simulink model "ASM"  (R2014a)
settings: Solver=ode45  StartTime=0.0  StopTime=30  FixedStep=0.002  MaxStep=0.2e-3  RelTol=1e-3
PreLoadFcn:
  | ASM_init
model workspace: external: MATLAB File /Users/Pascal/Documents/Beuth Hochschule/EPE-MES/04_Simulation/ASM/ASM_init.m (data not in the file)
values from neighbouring files (symbols this model uses):
  J = 0.0006    [ASM_init.m]    (also in parameter.mat)
  LR_plus = 0.89737    [ASM_init.m]    (also in parameter.mat)
  Lsigma_plus = 0.12968    [ASM_init.m]    (also in parameter.mat)
  MLast = 2    [ASM_init.m]    (also in parameter.mat = 20)
  MLast1 = 3.8    [ASM_init.m]
  PsiR_plus = 0.64521    [ASM_init.m]    (also in parameter.mat)
  RR_plus = 26.3    [ASM_init.m]    (also in parameter.mat)
  Rreib = 0.00138    [ASM_init.m]    (also in parameter.mat = 0.16)
  Rs = 32.65    [ASM_init.m]    (also in parameter.mat)
  wSoll = 500    [ASM_init.m]
  wSoll2 = 200    [ASM_init.m]
libraries: powerlib x25, simulink x3
settings Model: SimulationMode=accelerator  Creator=Pascal  LastModifiedBy=Pascal
settings DataIOCC: ExternalInput=parameter.mat  FinalStateName=ASM_state  InitialState=ASM_state  LimitDataPoints=off  SaveCompleteFinalSimState=on  SaveOutput=off
settings HardwareCC: ProdBitPerChar=16  ProdBitPerInt=16  ProdBitPerPointer=16  ProdLargestAtomicInteger=Integer  ProdIntDivRoundTo=Zero  ProdEndianess=LittleEndian  ProdWordSize=16  ProdHWDeviceType=Texas Instruments->C2000

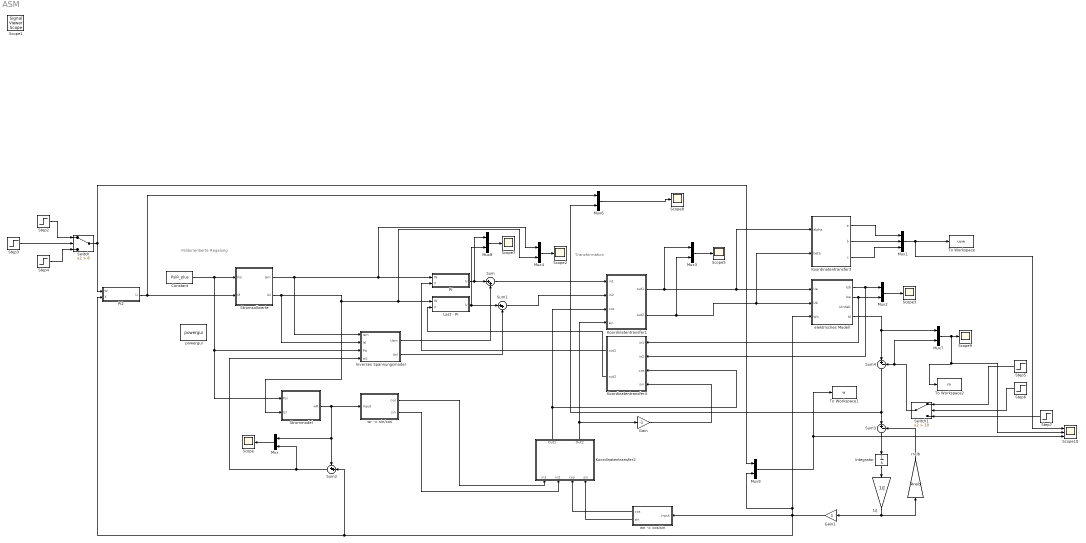
== system ASM ==
  note: Transformation
  note: Feldorientierte Regelung
  1/J : Gain  Gain=1/J
  Constant : Constant  Value=PsiR_plus
  Gain : Gain  Gain=-1
  Gain1 : Gain
  Integrator : Integrator
  "Inverses Spannungsmodel " : Subsystem
  Koordinatentransfer1 : Subsystem
  Koordinatentransfer2 : Subsystem
  Koordinatentransfer3 : Subsystem
  Koordinatentransfer4 : Subsystem
  Last - PI : Subsystem
  Mux{,2..4,6..9} (8 alike) : Mux  Inputs=2
  Mux1 : Mux  Inputs=3
  PI : Subsystem
  PI2 : Subsystem
  Scope{,2..3,5,7..9} (7 alike) : Scope
      Scope settings: ShowLegends=on  TimeRange=1  YMin=200  YMax=1500  SaveName=ScopeData6
      Scope2 settings: ShowLegends=on  TimeRange=4  YMin=-0.325  YMax=0.15
      Scope3 settings: ShowLegends=on  YMin=5000  YMax=70000  SaveName=ScopeData9
      Scope5 settings: YMin=-900  YMax=900
      Scope7 settings: ShowLegends=on  TimeRange=4  YMin=120  YMax=330  SaveName=ScopeData3
      Scope8 settings: ShowLegends=on  YMin=1  YMax=1.8  SaveName=ScopeData4
      Scope9 settings: ShowLegends=on  YMin=1.38778e-17  YMax=0.3  SaveName=ScopeData7
  Scope10 : Scope  NumInputPorts=3
      settings: ShowLegends=on  TimeRange=4  YMin=-1500~0~1350  YMax=1500~2~1420  SaveName=ScopeData10
  Step2 : Step  Before=1350  After=wSoll  SampleTime=0
  Step3 : Step  Time=8  After=200  SampleTime=0
  Step4 : Step  Time=3  Before=1350  After=wSoll2  SampleTime=0
  Step5 : Step  Time=4  After=MLast  SampleTime=0
  Step6 : Step  Time=10  After=200  SampleTime=0
  Step7 : Step  Time=3  After=MLast1  SampleTime=0
  "Strommodel " : Subsystem
  Stromsollwerte : Subsystem
  Sum : Sum  Inputs=|++
  Sum1 : Sum  Inputs=|++
  Sum2 : Sum  Inputs=++|
  Sum3 : Sum  Inputs=|+-
  Sum4 : Sum  Inputs=|+-
  Switch : Switch  Criteria=u2 > Threshold  Threshold=8
  Switch1 : Switch  Criteria=u2 > Threshold  Threshold=10
  To Workspace : ToWorkspace  VariableName=uvw  SampleTime=-1
  To Workspace1 : ToWorkspace  VariableName=w  SampleTime=-1
  To Workspace2 : ToWorkspace  VariableName=m  SampleTime=-1
  elektrisches Modell : Subsystem
  powergui : powerlib/powergui  Priority=1  SimulationMode=Continuous  SolverType=Tustin  SampleTime=50e-6  frequency=60  SPID=off  DisableSnubberDevices=off  DisableRonSwitches=off  DisableVfSwitches=off  SwTol=0  Interpol=off  DisplayEquations=off  Ts=0  methode=off  frequencyindice=0  Pbase=100e6  ErrMax=1e-4  Iterations=50  UnitsV=kV  UnitsW=MW  FunctionMessages=off  echomessages=off  HookPort=off  EnableUseOfTLC=off  x0status=blocks  RestoreLinks=warning  ResistiveCurrentMeasurement=off  Frange=[0:2:500]  Ylog=off  Xlog=on  ShowGrid=off  save=off  variable=ZData  structure=0  ZoomFFT=off  StartTime=0.0  cycles=1  DisplayStyle=1  fundamental=60  FreqAxis=off  MaxFrequency=1000  frequencyindicesteady=1  RmsSteady=1  display=off
  rreib : Gain  Gain=Rreib
  "wn -> cos/sin" : Subsystem
  "wr -> sin/cos" : Subsystem
  Scope1 : SignalViewerScope  IOType=viewer  ZoomMode=xonly  RefreshTime=0.035000
  wires:
  Mux2/1 -> Scope3/1
  Koordinatentransfer2/2(Out2) -> Gain/1, Koordinatentransfer1/4(sin)
  "wn -> cos/sin"/1(cos) -> Koordinatentransfer2/3(cos)
  "Strommodel "/1(wR) -> Sum2/1, Mux/1, "wr -> sin/cos"/1(Input)
  "wn -> cos/sin"/2(sin) -> Koordinatentransfer2/4("sin ")
  "wr -> sin/cos"/1(cos) -> Koordinatentransfer2/1(in1)
  Sum2/1 -> Mux/2, "Inverses Spannungsmodel "/4(wS)
  PI/1(U) -> Mux8/1, Sum/1
  Koordinatentransfer2/1(Out1) -> Koordinatentransfer1/3(cos), Koordinatentransfer4/3(cos)
  "wr -> sin/cos"/2(sin) -> Koordinatentransfer2/2(in2)
  Last - PI/1(U) -> Mux8/2, Sum1/1
  elektrisches Modell/1(Isb) -> Koordinatentransfer4/2(in2), Mux2/1
  elektrisches Modell/2(Isa) -> Koordinatentransfer4/1(in1), Mux2/2
  Koordinatentransfer3/2(b) -> Mux1/2
  Koordinatentransfer3/1(a) -> Mux1/1
  Koordinatentransfer3/3(c) -> Mux1/3
  1/J/1 -> rreib/1, Gain1/1
  Mux3/1 -> Scope5/1
  Constant/1 -> "Strommodel "/1(Psi), "Inverses Spannungsmodel "/3(Psi), Stromsollwerte/1(Psi)
  Gain/1 -> Koordinatentransfer4/4(sin)
  Sum3/1 -> Integrator/1
  rreib/1 -> Sum3/2
  Integrator/1 -> 1/J/1
  Sum4/1 -> Mux6/2, Sum3/1
  Mux6/1 -> Scope8/1
  Mux/1 -> Scope/1
  Mux7/1 -> To Workspace2/1, Scope10/2, Scope9/1
  elektrisches Modell/4(M) -> Mux7/1, Sum4/1
  Switch1/1 -> Mux7/2, Sum4/2
  Stromsollwerte/1(Ism) -> Mux4/1, PI/1(W), "Inverses Spannungsmodel "/1(Ism)
  Stromsollwerte/2(Isl) -> "Inverses Spannungsmodel "/2(Isl), "Strommodel "/2(Isl), Mux4/2, Last - PI/1(W)
  Koordinatentransfer4/2(out2) -> Last - PI/2(X)
  Koordinatentransfer4/1(out1) -> PI/2(X)
  Step2/1 -> Switch/1
  Mux1/1 -> Scope10/1, To Workspace/1
  Mux9/1 -> Scope10/3, To Workspace1/1
  Switch/1 -> PI2/1(W), Mux9/1
  Step4/1 -> Switch/3
  Step3/1 -> Switch/2
  Koordinatentransfer1/2(out2) -> Mux3/2, elektrisches Modell/2(Ub), Koordinatentransfer3/2(beta)
  Koordinatentransfer1/1(out1) -> elektrisches Modell/1(Ua), Koordinatentransfer3/1(alpha), Mux3/1
  Mux8/1 -> Scope7/1
  Mux4/1 -> Scope2/1
  "Inverses Spannungsmodel "/1(Usm) -> Sum/2
  "Inverses Spannungsmodel "/2(Usl) -> Sum1/2
  Sum/1 -> Koordinatentransfer1/1(in1)
  Sum1/1 -> Koordinatentransfer1/2(in2)
  Gain1/1 -> Mux9/2, elektrisches Modell/3(Wn), "wn -> cos/sin"/1(Input), PI2/2(X), Sum2/2
  PI2/1(U) -> Stromsollwerte/2(M), Mux6/1
  Step5/1 -> Switch1/1
  Step7/1 -> Switch1/3
  Step6/1 -> Switch1/2

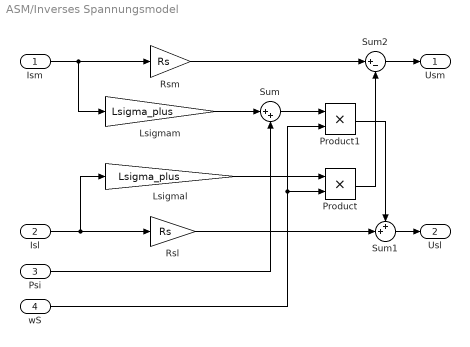
== system ASM/Inverses Spannungsmodel  ==
  Ism : Inport
  Isl : Inport  Port=2
  Psi : Inport  Port=3
  wS : Inport  Port=4
  Lsigmal : Gain  Gain=Lsigma_plus
  Lsigmam : Gain  Gain=Lsigma_plus
  Product : Product
  Product1 : Product
  Rsl : Gain  Gain=Rs
  Rsm : Gain  Gain=Rs
  Sum : Sum  Inputs=|++
  Sum1 : Sum  Inputs=++|
  Sum2 : Sum  Inputs=|+-
  Usm : Outport
  Usl : Outport  Port=2
  wires:
  Lsigmam/1 -> Sum/1
  Ism/1 -> Rsm/1, Lsigmam/1
  Isl/1 -> Rsl/1, Lsigmal/1
  Sum2/1 -> Usm/1
  Sum1/1 -> Usl/1
  Sum/1 -> Product1/1
  wS/1 -> Product1/2, Product/2
  Lsigmal/1 -> Product/1
  Psi/1 -> Sum/2
  Product1/1 -> Sum1/1
  Product/1 -> Sum2/2
  Rsm/1 -> Sum2/1
  Rsl/1 -> Sum1/2

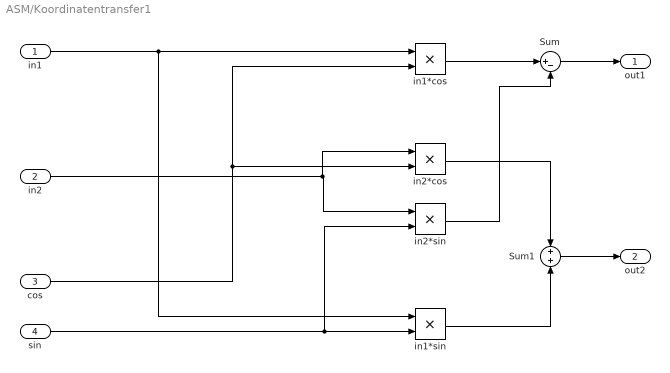
== system ASM/Koordinatentransfer1 ==
  in1 : Inport
  in2 : Inport  Port=2
  cos : Inport  Port=3
  sin : Inport  Port=4
  Sum : Sum  Inputs=|+-
  Sum1 : Sum
  in1*cos : Product
  in1*sin : Product
  in2*cos : Product
  in2*sin : Product
  out1 : Outport
  out2 : Outport  Port=2
  wires:
  in1/1 -> in1*sin/1, in1*cos/1
  cos/1 -> in2*cos/2, in1*cos/2
  sin/1 -> in2*sin/2, in1*sin/2
  in2/1 -> in2*cos/1, in2*sin/1
  in1*sin/1 -> Sum1/2
  in2*cos/1 -> Sum1/1
  in2*sin/1 -> Sum/2
  in1*cos/1 -> Sum/1
  Sum/1 -> out1/1
  Sum1/1 -> out2/1

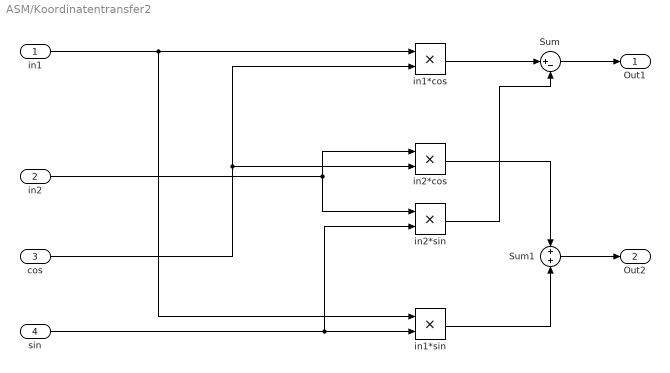
== system ASM/Koordinatentransfer2 ==
  in1 : Inport
  in2 : Inport  Port=2
  cos : Inport  Port=3
  "sin " : Inport  Port=4
  Sum : Sum  Inputs=|+-
  Sum1 : Sum
  in1*cos : Product
  in1*sin : Product
  in2*cos : Product
  in2*sin : Product
  Out1 : Outport
  Out2 : Outport  Port=2
  wires:
  in1/1 -> in1*sin/1, in1*cos/1
  cos/1 -> in2*cos/2, in1*cos/2
  "sin "/1 -> in2*sin/2, in1*sin/2
  in2/1 -> in2*cos/1, in2*sin/1
  in1*sin/1 -> Sum1/2
  in2*cos/1 -> Sum1/1
  in2*sin/1 -> Sum/2
  in1*cos/1 -> Sum/1
  Sum/1 -> Out1/1
  Sum1/1 -> Out2/1

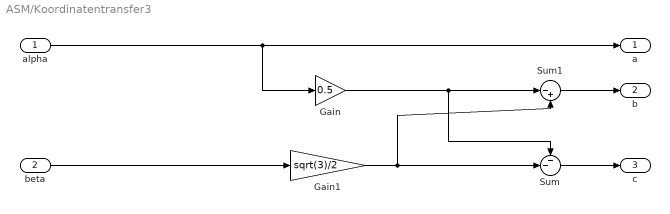
== system ASM/Koordinatentransfer3 ==
  alpha : Inport
  beta : Inport  Port=2
  Gain : Gain  Gain=0.5
  Gain1 : Gain  Gain=sqrt(3)/2
  Sum : Sum  Inputs=--|
  Sum1 : Sum  Inputs=|-+
  a : Outport
  b : Outport  Port=2
  c : Outport  Port=3
  wires:
  alpha/1 -> Gain/1, a/1
  Sum1/1 -> b/1
  Gain/1 -> Sum/1, Sum1/1
  Gain1/1 -> Sum/2, Sum1/2
  beta/1 -> Gain1/1
  Sum/1 -> c/1

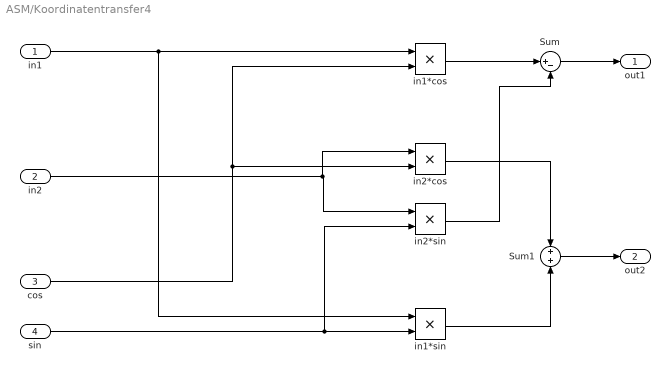
== system ASM/Koordinatentransfer4 ==
  in1 : Inport
  in2 : Inport  Port=2
  cos : Inport  Port=3
  sin : Inport  Port=4
  Sum : Sum  Inputs=|+-
  Sum1 : Sum
  in1*cos : Product
  in1*sin : Product
  in2*cos : Product
  in2*sin : Product
  out1 : Outport
  out2 : Outport  Port=2
  wires:
  in1/1 -> in1*sin/1, in1*cos/1
  cos/1 -> in2*cos/2, in1*cos/2
  sin/1 -> in2*sin/2, in1*sin/2
  in2/1 -> in2*cos/1, in2*sin/1
  in1*sin/1 -> Sum1/2
  in2*cos/1 -> Sum1/1
  in2*sin/1 -> Sum/2
  in1*cos/1 -> Sum/1
  Sum/1 -> out1/1
  Sum1/1 -> out2/1

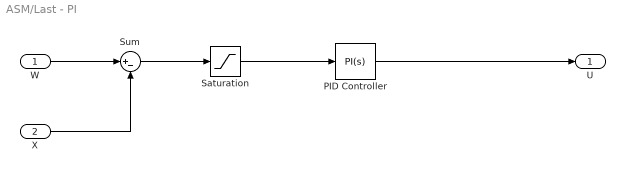
== system ASM/Last - PI ==
  W : Inport
  X : Inport  Port=2
  PID Controller : simulink/Continuous/PID Controller  Controller=PI  TimeDomain=Continuous-time  SampleTime=1  IntegratorMethod=Forward Euler  FilterMethod=Forward Euler  Form=Parallel  P=3.02729379594108  I=59.0597737641669  D=0.0225096512911581  N=2097943.11620465  InitialConditionSource=internal  InitialConditionForIntegrator=0  InitialConditionForFilter=0  ExternalReset=none  LimitOutput=on  UpperSaturationLimit=325  LowerSaturationLimit=-325  LinearizeAsGain=off  AntiWindupMode=none  Kb=1  TrackingMode=off  Kt=1  PParamMin=[]  PParamMax=[]  IParamMin=[]  IParamMax=[]  DParamMin=[]  DParamMax=[]  NParamMin=[]  NParamMax=[]  KbParamMin=[]  KbParamMax=[]  KtParamMin=[]  KtParamMax=[]  POutMin=[]  POutMax=[]  IOutMin=[]  IOutMax=[]  DOutMin=[]  DOutMax=[]  NOutMin=[]  NOutMax=[]  KbOutMin=[]  KbOutMax=[]  KtOutMin=[]  KtOutMax=[]  IntegratorOutMin=[]  IntegratorOutMax=[]  FilterOutMin=[]  FilterOutMax=[]  SumOutMin=[]  SumOutMax=[]  SumI1OutMin=[]  SumI1OutMax=[]  SumI2OutMin=[]  SumI2OutMax=[]  SumI3OutMin=[]  SumI3OutMax=[]  SumDOutMin=[]  SumDOutMax=[]  SaturationOutMin=[]  SaturationOutMax=[]  IntegratorContinuousStateAttributes=''  IntegratorStateMustResolveToSignalObject=off  IntegratorRTWStateStorageClass=Auto  FilterContinuousStateAttributes=''  FilterStateMustResolveToSignalObject=off  FilterRTWStateStorageClass=Auto
  Saturation : Saturate  UpperLimit=3.8  LowerLimit=-3.8  LinearizeAsGain=off
  Sum : Sum  Inputs=|+-
  U : Outport
  wires:
  W/1 -> Sum/1
  X/1 -> Sum/2
  Sum/1 -> Saturation/1
  PID Controller/1 -> U/1
  Saturation/1 -> PID Controller/1

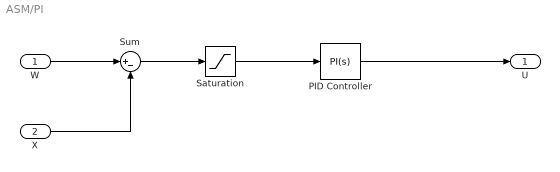
== system ASM/PI ==
  W : Inport
  X : Inport  Port=2
  PID Controller : simulink/Continuous/PID Controller  Controller=PI  TimeDomain=Continuous-time  SampleTime=1  IntegratorMethod=Forward Euler  FilterMethod=Forward Euler  Form=Parallel  P=3.02729379594108  I=59.0597737641669  D=0.0225096512911581  N=2097943.11620465  InitialConditionSource=internal  InitialConditionForIntegrator=0  InitialConditionForFilter=0  ExternalReset=none  LimitOutput=on  UpperSaturationLimit=325  LowerSaturationLimit=-325  LinearizeAsGain=off  AntiWindupMode=none  Kb=1  TrackingMode=off  Kt=1  PParamMin=[]  PParamMax=[]  IParamMin=[]  IParamMax=[]  DParamMin=[]  DParamMax=[]  NParamMin=[]  NParamMax=[]  KbParamMin=[]  KbParamMax=[]  KtParamMin=[]  KtParamMax=[]  POutMin=[]  POutMax=[]  IOutMin=[]  IOutMax=[]  DOutMin=[]  DOutMax=[]  NOutMin=[]  NOutMax=[]  KbOutMin=[]  KbOutMax=[]  KtOutMin=[]  KtOutMax=[]  IntegratorOutMin=[]  IntegratorOutMax=[]  FilterOutMin=[]  FilterOutMax=[]  SumOutMin=[]  SumOutMax=[]  SumI1OutMin=[]  SumI1OutMax=[]  SumI2OutMin=[]  SumI2OutMax=[]  SumI3OutMin=[]  SumI3OutMax=[]  SumDOutMin=[]  SumDOutMax=[]  SaturationOutMin=[]  SaturationOutMax=[]  IntegratorContinuousStateAttributes=''  IntegratorStateMustResolveToSignalObject=off  IntegratorRTWStateStorageClass=Auto  FilterContinuousStateAttributes=''  FilterStateMustResolveToSignalObject=off  FilterRTWStateStorageClass=Auto
  Saturation : Saturate  UpperLimit=3.8  LowerLimit=-3.8  LinearizeAsGain=off
  Sum : Sum  Inputs=|+-
  U : Outport
  wires:
  W/1 -> Sum/1
  X/1 -> Sum/2
  Sum/1 -> Saturation/1
  PID Controller/1 -> U/1
  Saturation/1 -> PID Controller/1

== system ASM/PI2 ==
  W : Inport
  X : Inport  Port=2
  PID Controller : simulink/Continuous/PID Controller  Controller=PI  TimeDomain=Continuous-time  SampleTime=1  IntegratorMethod=Forward Euler  FilterMethod=Forward Euler  Form=Parallel  P=0.0785257439463388  I=0.0278541269001317  D=0  N=1000  InitialConditionSource=internal  InitialConditionForIntegrator=0  InitialConditionForFilter=0  ExternalReset=none  LimitOutput=on  UpperSaturationLimit=3.4  LowerSaturationLimit=-3.4  LinearizeAsGain=off  AntiWindupMode=none  Kb=1  TrackingMode=off  Kt=1  PParamMin=[]  PParamMax=[]  IParamMin=[]  IParamMax=[]  DParamMin=[]  DParamMax=[]  NParamMin=[]  NParamMax=[]  KbParamMin=[]  KbParamMax=[]  KtParamMin=[]  KtParamMax=[]  POutMin=[]  POutMax=[]  IOutMin=[]  IOutMax=[]  DOutMin=[]  DOutMax=[]  NOutMin=[]  NOutMax=[]  KbOutMin=[]  KbOutMax=[]  KtOutMin=[]  KtOutMax=[]  IntegratorOutMin=[]  IntegratorOutMax=[]  FilterOutMin=[]  FilterOutMax=[]  SumOutMin=[]  SumOutMax=[]  SumI1OutMin=[]  SumI1OutMax=[]  SumI2OutMin=[]  SumI2OutMax=[]  SumI3OutMin=[]  SumI3OutMax=[]  SumDOutMin=[]  SumDOutMax=[]  SaturationOutMin=[]  SaturationOutMax=[]  IntegratorContinuousStateAttributes=''  IntegratorStateMustResolveToSignalObject=off  IntegratorRTWStateStorageClass=Auto  FilterContinuousStateAttributes=''  FilterStateMustResolveToSignalObject=off  FilterRTWStateStorageClass=Auto
  Sum : Sum  Inputs=|+-
  U : Outport
  wires:
  W/1 -> Sum/1
  X/1 -> Sum/2
  PID Controller/1 -> U/1
  Sum/1 -> PID Controller/1

== system ASM/Strommodel  ==
  Psi : Inport
  Isl : Inport  Port=2
  Divide : Product  Inputs=*/
  Rr : Gain  Gain=RR_plus
  wR : Outport
  wires:
  Rr/1 -> wR/1
  Divide/1 -> Rr/1
  Psi/1 -> Divide/2
  Isl/1 -> Divide/1

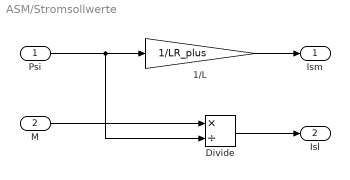
== system ASM/Stromsollwerte ==
  Psi : Inport
  M : Inport  Port=2
  1/L : Gain  Gain=1/LR_plus
  Divide : Product  Inputs=*/
  Ism : Outport  OutMax=1.8
  Isl : Outport  Port=2  OutMax=[1.8]
  wires:
  1/L/1 -> Ism/1
  Psi/1 -> Divide/2, 1/L/1
  Divide/1 -> Isl/1
  M/1 -> Divide/1

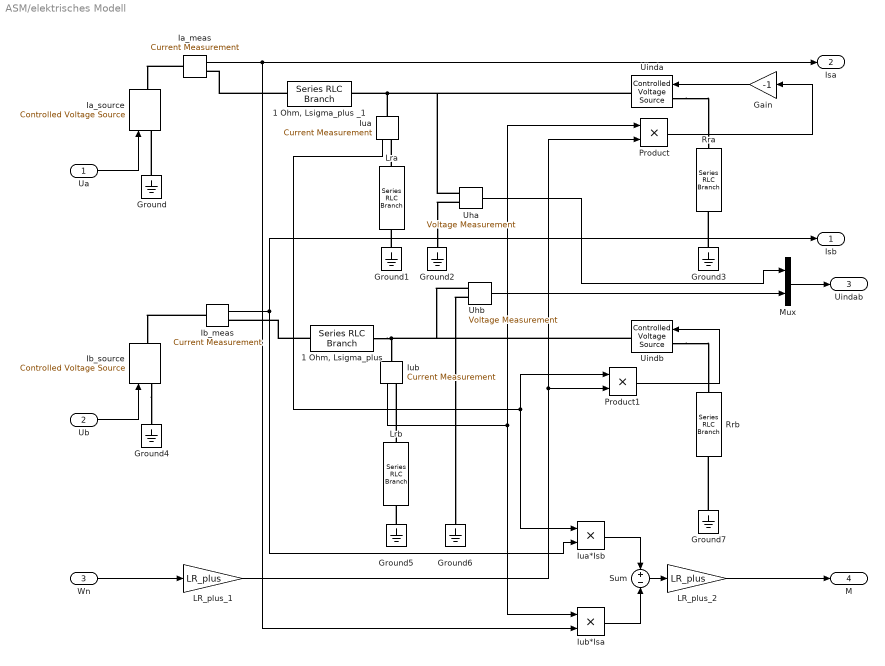
== system ASM/elektrisches Modell ==
  Ua : Inport
  Ub : Inport  Port=2
  Wn : Inport  Port=3
  "1 Ohm, Lsigma_plus" : powerlib/Elements/Series RLC Branch  LConnTagsString=__new0  RConnTagsString=__new0  BranchType=RL  Resistance=RR_plus  Inductance=Lsigma_plus  SetiL0=on  InitialCurrent=10  Capacitance=1e-6  Setx0=off  InitialVoltage=0  Measurements=None
  "1 Ohm, Lsigma_plus _1 " : powerlib/Elements/Series RLC Branch  LConnTagsString=__new0  RConnTagsString=__new0  BranchType=RL  Resistance=RR_plus  Inductance=Lsigma_plus  SetiL0=on  InitialCurrent=10  Capacitance=1e-6  Setx0=off  InitialVoltage=0  Measurements=None
  Gain : Gain  Gain=-1
  Ground{,1..7} (8 alike) : powerlib/Elements/Ground  LConnTagsString=a
  Ia_meas : powerlib/Measurements/Current Measurement  PhasorSimulation=off  OutputType=Complex  PSBequivalent=0
  Ia_source : powerlib/Electrical Sources/Controlled Voltage Source  Initialize=on  Source_Type=AC  Amplitude=0  Phase=0  Frequency=0  Measurements=None
  Ib_meas : powerlib/Measurements/Current Measurement  PhasorSimulation=off  OutputType=Complex  PSBequivalent=0
  Ib_source : powerlib/Electrical Sources/Controlled Voltage Source  Initialize=on  Source_Type=AC  Amplitude=0  Phase=0  Frequency=0  Measurements=None
  Iua : powerlib/Measurements/Current Measurement  PhasorSimulation=off  OutputType=Complex  PSBequivalent=0
  Iua*Isb : Product
  Iub : powerlib/Measurements/Current Measurement  PhasorSimulation=off  OutputType=Complex  PSBequivalent=0
  Iub*Isa : Product
  LR_plus_1 : Gain  Gain=LR_plus
  LR_plus_2 : Gain  Gain=LR_plus
  Lra : powerlib/Elements/Series RLC Branch  LConnTagsString=__new0  RConnTagsString=__new0  BranchType=L  Resistance=1  Inductance=LR_plus  SetiL0=on  InitialCurrent=10  Capacitance=1e-6  Setx0=off  InitialVoltage=0  Measurements=None
  Lrb : powerlib/Elements/Series RLC Branch  LConnTagsString=__new0  RConnTagsString=__new0  BranchType=L  Resistance=1  Inductance=LR_plus  SetiL0=on  InitialCurrent=10  Capacitance=1e-6  Setx0=off  InitialVoltage=0  Measurements=None
  Mux : Mux  Inputs=2
  Product : Product
  Product1 : Product
  Rra : powerlib/Elements/Series RLC Branch  LConnTagsString=__new0  RConnTagsString=__new0  BranchType=R  Resistance=RR_plus  Inductance=100e-3  SetiL0=off  InitialCurrent=0  Capacitance=1e-6  Setx0=off  InitialVoltage=0  Measurements=None
  Rrb : powerlib/Elements/Series RLC Branch  LConnTagsString=__new0  RConnTagsString=__new0  BranchType=R  Resistance=RR_plus  Inductance=100e-3  SetiL0=off  InitialCurrent=0  Capacitance=1e-6  Setx0=off  InitialVoltage=0  Measurements=None
  Sum : Sum  Inputs=+|-
  Uha : powerlib/Measurements/Voltage Measurement  PhasorSimulation=off  OutputType=Complex  PSBequivalent=0
  Uhb : powerlib/Measurements/Voltage Measurement  PhasorSimulation=off  OutputType=Complex  PSBequivalent=0
  Uinda : powerlib/Electrical Sources/Controlled Voltage Source  Initialize=on  Source_Type=AC  Amplitude=0  Phase=0  Frequency=0  Measurements=None
  Uindb : powerlib/Electrical Sources/Controlled Voltage Source  Initialize=on  Source_Type=AC  Amplitude=0  Phase=0  Frequency=0  Measurements=None
  Isb : Outport
  Isa : Outport  Port=2
  Uindab : Outport  Port=3
  M : Outport  Port=4
  wires:
  Ua/1 -> Ia_source/1
  Ia_meas/1 -> Iub*Isa/2, Isa/1
  Gain/1 -> Uinda/1
  Product/1 -> Gain/1
  Ub/1 -> Ib_source/1
  Ib_meas/1 -> Iua*Isb/2, Isb/1
  Uhb/1 -> Mux/2
  Uha/1 -> Mux/1
  Iub/1 -> Iub*Isa/1, Product/1
  Product1/1 -> Uindb/1
  Iua/1 -> Product1/1, Iua*Isb/1
  Wn/1 -> LR_plus_1/1
  LR_plus_1/1 -> Product/2, Product1/2
  Mux/1 -> Uindab/1
  Sum/1 -> LR_plus_2/1
  Iub*Isa/1 -> Sum/2
  Iua*Isb/1 -> Sum/1
  LR_plus_2/1 -> M/1
  connections:
  Ground/LConn1 -- Ia_source/LConn1
  Ia_meas/LConn1 -- Ia_source/RConn1
  "1 Ohm, Lsigma_plus _1 "/LConn1 -- Ia_meas/RConn1
  Iua/LConn1 -- Uha/LConn1 -- Uinda/RConn1 -- "1 Ohm, Lsigma_plus _1 "/RConn1
  Lra/LConn1 -- Iua/RConn1
  Ground1/LConn1 -- Lra/RConn1
  Uha/LConn2 -- Ground2/LConn1
  Uinda/LConn1 -- Rra/LConn1
  Ground3/LConn1 -- Rra/RConn1
  Ib_source/LConn1 -- Ground4/LConn1
  Ib_meas/LConn1 -- Ib_source/RConn1
  "1 Ohm, Lsigma_plus"/LConn1 -- Ib_meas/RConn1
  Lrb/LConn1 -- Iub/RConn1
  Ground5/LConn1 -- Lrb/RConn1
  Uhb/LConn2 -- Ground6/LConn1
  "1 Ohm, Lsigma_plus"/RConn1 -- Uindb/RConn1 -- Uhb/LConn1 -- Iub/LConn1
  Ground7/LConn1 -- Rrb/RConn1
  Uindb/LConn1 -- Rrb/LConn1

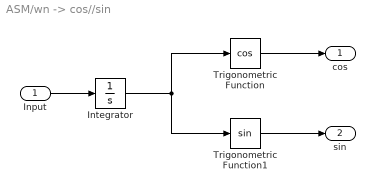
== system ASM/wn -> cos//sin ==
  Input : Inport
  Integrator : Integrator
  Trigonometric Function : Trigonometry  Operator=cos
  Trigonometric Function1 : Trigonometry
  cos : Outport
  sin : Outport  Port=2
  wires:
  Trigonometric Function/1 -> cos/1
  Trigonometric Function1/1 -> sin/1
  Integrator/1 -> Trigonometric Function/1, Trigonometric Function1/1
  Input/1 -> Integrator/1

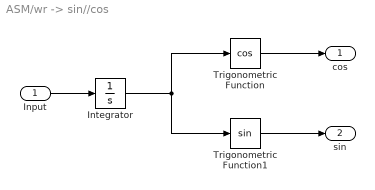
== system ASM/wr -> sin//cos ==
  Input : Inport
  Integrator : Integrator
  Trigonometric Function : Trigonometry  Operator=cos
  Trigonometric Function1 : Trigonometry
  cos : Outport
  sin : Outport  Port=2
  wires:
  Trigonometric Function/1 -> cos/1
  Trigonometric Function1/1 -> sin/1
  Integrator/1 -> Trigonometric Function/1, Trigonometric Function1/1
  Input/1 -> Integrator/1
